simulink model "UserPowerTrain"  (R2025a)
settings: Solver=ode1  StartTime=0.0  StopTime=inf  FixedStep=0.001  RelTol=1e-3  EnableMultiTasking=on
undefined symbols (not defined in the file): DiscIntNeverNeededParam
libraries: CarMaker4SL x7
(part 2 of 3)

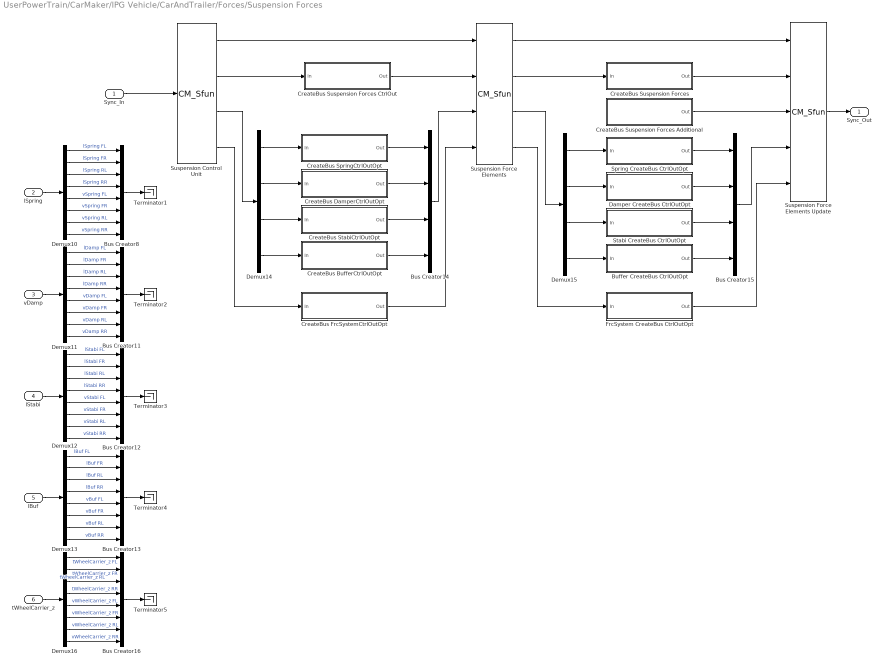
== system UserPowerTrain/CarMaker/IPG Vehicle/CarAndTrailer/Forces/Suspension Forces ==
  Sync_In : Inport
  lSpring : Inport  Port=2
  vDamp : Inport  Port=3
  lStabi : Inport  Port=4
  lBuf : Inport  Port=5
  tWheelCarrier_z : Inport  Port=6
  Buffer CreateBus CtrlOutOpt : Subsystem
  Bus Creator{8,11..13,16} (5 alike) : BusCreator  Inputs=8
  Bus Creator14 : BusCreator  Inputs=4
  Bus Creator15 : BusCreator  Inputs=4
  CreateBus BufferCtrlOutOpt : Subsystem
  CreateBus DamperCtrlOutOpt : Subsystem
  CreateBus FrcSystemCtrlOutOpt : Subsystem
  CreateBus SpringCtrlOutOpt : Subsystem
  CreateBus StabiCtrlOutOpt : Subsystem
  CreateBus Suspension Forces : Subsystem
  CreateBus Suspension Forces Additional : Subsystem
  CreateBus Suspension Forces CtrlOut : Subsystem
  Damper CreateBus CtrlOutOpt : Subsystem
  Demux{10..13,16} (5 alike) : Demux  Outputs=8
      settings: DisplayOption=none
  Demux14 : Demux
      settings: DisplayOption=none
  Demux15 : Demux
      settings: DisplayOption=none
  FrcSystem CreateBus CtrlOutOpt : Subsystem
  Spring CreateBus CtrlOutOpt : Subsystem
  Stabi CreateBus CtrlOutOpt : Subsystem
  Suspension Control Unit : S-Function  FunctionName=CM_Sfun  Parameters='ForcesSuspControl'  SFunctionDeploymentMode=off  EnableBusSupport=off
  Suspension Force Elements : S-Function  FunctionName=CM_Sfun  Parameters='ForcesSusp'  SFunctionDeploymentMode=off  EnableBusSupport=off
  Suspension Force Elements Update : S-Function  FunctionName=CM_Sfun  Parameters='ForcesSuspUpd'  SFunctionDeploymentMode=off  EnableBusSupport=off
  Terminator{1..5} (5 alike) : Terminator
  Sync_Out : Outport  VectorParamsAs1DForOutWhenUnconnected=off
  wires:
  Sync_In/1 -> Suspension Control Unit/1
  Suspension Control Unit/1 -> Suspension Force Elements/1
  Suspension Force Elements/1 -> Suspension Force Elements Update/1
  Suspension Force Elements Update/1 -> Sync_Out/1
  Demux13/4 -> Bus Creator13/4  "lBuf RR"
  Demux11/2 -> Bus Creator11/2  "lDamp FR"
  Demux13/8 -> Bus Creator13/8  "vBuf RR"
  Demux10/3 -> Bus Creator8/3  "lSpring RL"
  Demux10/1 -> Bus Creator8/1  "lSpring FL"
  vDamp/1 -> Demux11/1
  Demux13/2 -> Bus Creator13/2  "lBuf FR"
  Demux10/5 -> Bus Creator8/5  "vSpring FL"
  Bus Creator12/1 -> Terminator3/1
  Demux12/7 -> Bus Creator12/7  "vStabi RL"
  Demux10/4 -> Bus Creator8/4  "lSpring RR"
  Demux12/2 -> Bus Creator12/2  "lStabi FR"
  Demux11/5 -> Bus Creator11/5  "vDamp FL"
  Demux10/8 -> Bus Creator8/8  "vSpring RR"
  Demux12/1 -> Bus Creator12/1  "lStabi FL"
  Demux12/3 -> Bus Creator12/3  "lStabi RL"
  Demux11/6 -> Bus Creator11/6  "vDamp FR"
  lSpring/1 -> Demux10/1
  lBuf/1 -> Demux13/1
  Demux12/4 -> Bus Creator12/4  "lStabi RR"
  Bus Creator13/1 -> Terminator4/1
  Demux13/7 -> Bus Creator13/7  "vBuf RL"
  Demux12/8 -> Bus Creator12/8  "vStabi RR"
  Demux10/7 -> Bus Creator8/7  "vSpring RL"
  Demux11/8 -> Bus Creator11/8  "vDamp RR"
  Demux12/6 -> Bus Creator12/6  "vStabi FR"
  Demux11/1 -> Bus Creator11/1  "lDamp FL"
  Demux11/7 -> Bus Creator11/7  "vDamp RL"
  lStabi/1 -> Demux12/1
  Demux12/5 -> Bus Creator12/5  "vStabi FL"
  Bus Creator8/1 -> Terminator1/1
  Bus Creator11/1 -> Terminator2/1
  Demux13/1 -> Bus Creator13/1  "lBuf FL"
  Demux13/6 -> Bus Creator13/6  "vBuf FR"
  Demux11/4 -> Bus Creator11/4  "lDamp RR"
  Demux13/5 -> Bus Creator13/5  "vBuf FL"
  Demux10/6 -> Bus Creator8/6  "vSpring FR"
  Demux11/3 -> Bus Creator11/3  "lDamp RL"
  Demux10/2 -> Bus Creator8/2  "lSpring FR"
  Demux13/3 -> Bus Creator13/3  "lBuf RL"
  Suspension Force Elements/4 -> FrcSystem CreateBus CtrlOutOpt/1(In)
  FrcSystem CreateBus CtrlOutOpt/1(Out) -> Suspension Force Elements Update/5
  CreateBus SpringCtrlOutOpt/1(Out) -> Bus Creator14/1
  Demux14/1 -> CreateBus SpringCtrlOutOpt/1(In)
  Demux14/2 -> CreateBus DamperCtrlOutOpt/1(In)
  CreateBus DamperCtrlOutOpt/1(Out) -> Bus Creator14/2
  Demux14/3 -> CreateBus StabiCtrlOutOpt/1(In)
  CreateBus StabiCtrlOutOpt/1(Out) -> Bus Creator14/3
  CreateBus BufferCtrlOutOpt/1(Out) -> Bus Creator14/4
  Demux14/4 -> CreateBus BufferCtrlOutOpt/1(In)
  Demux15/4 -> Buffer CreateBus CtrlOutOpt/1(In)
  Buffer CreateBus CtrlOutOpt/1(Out) -> Bus Creator15/4
  Demux15/3 -> Stabi CreateBus CtrlOutOpt/1(In)
  Stabi CreateBus CtrlOutOpt/1(Out) -> Bus Creator15/3
  Demux15/2 -> Damper CreateBus CtrlOutOpt/1(In)
  Damper CreateBus CtrlOutOpt/1(Out) -> Bus Creator15/2
  Demux15/1 -> Spring CreateBus CtrlOutOpt/1(In)
  Spring CreateBus CtrlOutOpt/1(Out) -> Bus Creator15/1
  Suspension Force Elements/3 -> Demux15/1
  Bus Creator15/1 -> Suspension Force Elements Update/4
  Demux16/1 -> Bus Creator16/1  "tWheelCarrier_z FL"
  Demux16/6 -> Bus Creator16/6  "vWheelCarrier_z FR"
  Bus Creator16/1 -> Terminator5/1
  Demux16/2 -> Bus Creator16/2  "tWheelCarrier_z FR"
  Demux16/4 -> Bus Creator16/4  "tWheelCarrier_z RR"
  Demux16/8 -> Bus Creator16/8  "vWheelCarrier_z RR"
  Demux16/7 -> Bus Creator16/7  "vWheelCarrier_z RL"
  Demux16/3 -> Bus Creator16/3  "tWheelCarrier_z RL"
  Demux16/5 -> Bus Creator16/5  "vWheelCarrier_z FL"
  tWheelCarrier_z/1 -> Demux16/1
  CreateBus Suspension Forces Additional/1(Out) -> Suspension Force Elements Update/3
  Suspension Force Elements/2 -> CreateBus Suspension Forces/1(In)
  CreateBus Suspension Forces/1(Out) -> Suspension Force Elements Update/2
  Suspension Control Unit/2 -> CreateBus Suspension Forces CtrlOut/1(In)
  Suspension Control Unit/3 -> Demux14/1
  Suspension Control Unit/4 -> CreateBus FrcSystemCtrlOutOpt/1(In)
  CreateBus FrcSystemCtrlOutOpt/1(Out) -> Suspension Force Elements/4
  Bus Creator14/1 -> Suspension Force Elements/3
  CreateBus Suspension Forces CtrlOut/1(Out) -> Suspension Force Elements/2

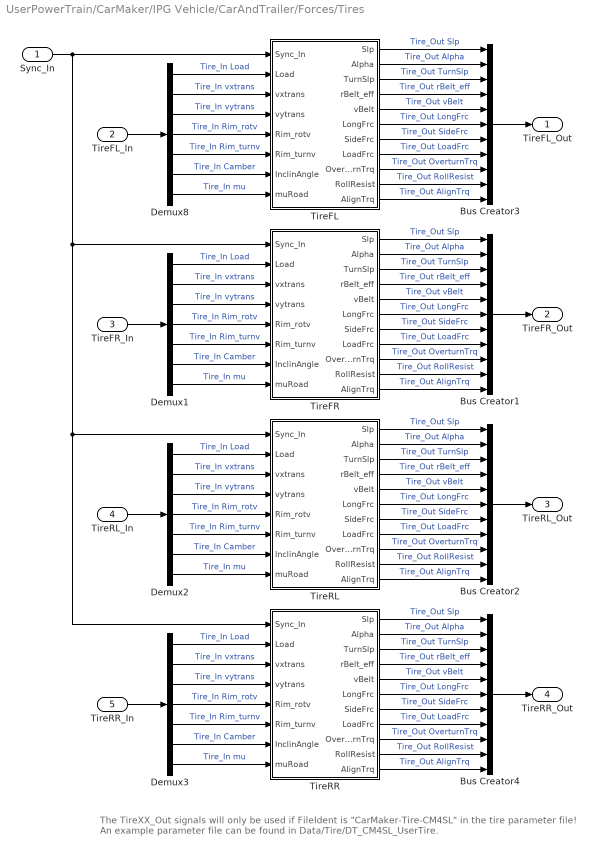
== system UserPowerTrain/CarMaker/IPG Vehicle/CarAndTrailer/Forces/Tires ==
  note: The TireXX_Out signals will only be used if FileIdent is "CarMaker-Tire-CM4SL" in the tire parameter file!
      | An example parameter file can be found in Data/Tire/DT_CM4SL_UserTire.
  Sync_In : Inport
  TireFL_In : Inport  Port=2
  TireFR_In : Inport  Port=3
  TireRL_In : Inport  Port=4
  TireRR_In : Inport  Port=5
  Bus Creator{1..4} (4 alike) : BusCreator  Inputs=11
  Demux{1..3,8} (4 alike) : Demux  Outputs=7
      settings: DisplayOption=none
  TireFL : Subsystem
  TireFR : Subsystem
  TireRL : Subsystem
  TireRR : Subsystem
  TireFL_Out : Outport  VectorParamsAs1DForOutWhenUnconnected=off
  TireFR_Out : Outport  Port=2  VectorParamsAs1DForOutWhenUnconnected=off
  TireRL_Out : Outport  Port=3  VectorParamsAs1DForOutWhenUnconnected=off
  TireRR_Out : Outport  Port=4  VectorParamsAs1DForOutWhenUnconnected=off
  wires:
  Sync_In/1 -> TireRR/1(Sync_In), TireRL/1(Sync_In), TireFR/1(Sync_In), TireFL/1(Sync_In)
  Bus Creator4/1 -> TireRR_Out/1
  Bus Creator2/1 -> TireRL_Out/1
  Bus Creator1/1 -> TireFR_Out/1
  Demux3/5 -> TireRR/6(Rim_turnv)  "Tire_In Rim_turnv"
  Demux3/4 -> TireRR/5(Rim_rotv)  "Tire_In Rim_rotv"
  Demux3/1 -> TireRR/2(Load)  "Tire_In Load"
  Demux3/7 -> TireRR/8(muRoad)  "Tire_In mu"
  Demux3/6 -> TireRR/7(InclinAngle)  "Tire_In Camber"
  Demux3/2 -> TireRR/3(vxtrans)  "Tire_In vxtrans"
  Demux3/3 -> TireRR/4(vytrans)  "Tire_In vytrans"
  TireRR/11(AlignTrq) -> Bus Creator4/11  "Tire_Out AlignTrq"
  TireRR/10(RollResist) -> Bus Creator4/10  "Tire_Out RollResist"
  TireRR/9(OverturnTrq) -> Bus Creator4/9  "Tire_Out OverturnTrq"
  TireRR/8(LoadFrc) -> Bus Creator4/8  "Tire_Out LoadFrc"
  TireRR/7(SideFrc) -> Bus Creator4/7  "Tire_Out SideFrc"
  TireRR/6(LongFrc) -> Bus Creator4/6  "Tire_Out LongFrc"
  TireRR/5(vBelt) -> Bus Creator4/5  "Tire_Out vBelt"
  TireRR/4(rBelt_eff) -> Bus Creator4/4  "Tire_Out rBelt_eff"
  TireRR/3(TurnSlp) -> Bus Creator4/3  "Tire_Out TurnSlp"
  TireRR/1(Slp) -> Bus Creator4/1  "Tire_Out Slp"
  TireRR/2(Alpha) -> Bus Creator4/2  "Tire_Out Alpha"
  Demux2/5 -> TireRL/6(Rim_turnv)  "Tire_In Rim_turnv"
  Demux2/4 -> TireRL/5(Rim_rotv)  "Tire_In Rim_rotv"
  Demux2/1 -> TireRL/2(Load)  "Tire_In Load"
  Demux2/7 -> TireRL/8(muRoad)  "Tire_In mu"
  Demux2/6 -> TireRL/7(InclinAngle)  "Tire_In Camber"
  Demux2/2 -> TireRL/3(vxtrans)  "Tire_In vxtrans"
  Demux2/3 -> TireRL/4(vytrans)  "Tire_In vytrans"
  TireRL/11(AlignTrq) -> Bus Creator2/11  "Tire_Out AlignTrq"
  TireRL/10(RollResist) -> Bus Creator2/10  "Tire_Out RollResist"
  TireRL/9(OverturnTrq) -> Bus Creator2/9  "Tire_Out OverturnTrq"
  TireRL/8(LoadFrc) -> Bus Creator2/8  "Tire_Out LoadFrc"
  TireRL/7(SideFrc) -> Bus Creator2/7  "Tire_Out SideFrc"
  TireRL/6(LongFrc) -> Bus Creator2/6  "Tire_Out LongFrc"
  TireRL/5(vBelt) -> Bus Creator2/5  "Tire_Out vBelt"
  TireRL/4(rBelt_eff) -> Bus Creator2/4  "Tire_Out rBelt_eff"
  TireRL/3(TurnSlp) -> Bus Creator2/3  "Tire_Out TurnSlp"
  TireRL/1(Slp) -> Bus Creator2/1  "Tire_Out Slp"
  TireRL/2(Alpha) -> Bus Creator2/2  "Tire_Out Alpha"
  Demux1/5 -> TireFR/6(Rim_turnv)  "Tire_In Rim_turnv"
  Demux1/4 -> TireFR/5(Rim_rotv)  "Tire_In Rim_rotv"
  Demux1/1 -> TireFR/2(Load)  "Tire_In Load"
  Demux1/7 -> TireFR/8(muRoad)  "Tire_In mu"
  Demux1/6 -> TireFR/7(InclinAngle)  "Tire_In Camber"
  Demux1/2 -> TireFR/3(vxtrans)  "Tire_In vxtrans"
  Demux1/3 -> TireFR/4(vytrans)  "Tire_In vytrans"
  TireFR/11(AlignTrq) -> Bus Creator1/11  "Tire_Out AlignTrq"
  TireFR/10(RollResist) -> Bus Creator1/10  "Tire_Out RollResist"
  TireFR/9(OverturnTrq) -> Bus Creator1/9  "Tire_Out OverturnTrq"
  TireFR/8(LoadFrc) -> Bus Creator1/8  "Tire_Out LoadFrc"
  TireFR/7(SideFrc) -> Bus Creator1/7  "Tire_Out SideFrc"
  TireFR/6(LongFrc) -> Bus Creator1/6  "Tire_Out LongFrc"
  TireFR/5(vBelt) -> Bus Creator1/5  "Tire_Out vBelt"
  TireFR/4(rBelt_eff) -> Bus Creator1/4  "Tire_Out rBelt_eff"
  TireFR/3(TurnSlp) -> Bus Creator1/3  "Tire_Out TurnSlp"
  TireFR/1(Slp) -> Bus Creator1/1  "Tire_Out Slp"
  TireFR/2(Alpha) -> Bus Creator1/2  "Tire_Out Alpha"
  Demux8/5 -> TireFL/6(Rim_turnv)  "Tire_In Rim_turnv"
  Demux8/4 -> TireFL/5(Rim_rotv)  "Tire_In Rim_rotv"
  TireFL_In/1 -> Demux8/1
  Demux8/1 -> TireFL/2(Load)  "Tire_In Load"
  Demux8/7 -> TireFL/8(muRoad)  "Tire_In mu"
  Demux8/6 -> TireFL/7(InclinAngle)  "Tire_In Camber"
  Demux8/2 -> TireFL/3(vxtrans)  "Tire_In vxtrans"
  Demux8/3 -> TireFL/4(vytrans)  "Tire_In vytrans"
  TireFL/11(AlignTrq) -> Bus Creator3/11  "Tire_Out AlignTrq"
  TireFL/10(RollResist) -> Bus Creator3/10  "Tire_Out RollResist"
  TireFL/9(OverturnTrq) -> Bus Creator3/9  "Tire_Out OverturnTrq"
  TireFL/8(LoadFrc) -> Bus Creator3/8  "Tire_Out LoadFrc"
  TireFL/7(SideFrc) -> Bus Creator3/7  "Tire_Out SideFrc"
  TireFL/6(LongFrc) -> Bus Creator3/6  "Tire_Out LongFrc"
  TireFL/5(vBelt) -> Bus Creator3/5  "Tire_Out vBelt"
  TireFL/4(rBelt_eff) -> Bus Creator3/4  "Tire_Out rBelt_eff"
  TireFL/3(TurnSlp) -> Bus Creator3/3  "Tire_Out TurnSlp"
  TireFL/1(Slp) -> Bus Creator3/1  "Tire_Out Slp"
  TireFL/2(Alpha) -> Bus Creator3/2  "Tire_Out Alpha"
  Bus Creator3/1 -> TireFL_Out/1
  TireFR_In/1 -> Demux1/1
  TireRL_In/1 -> Demux2/1
  TireRR_In/1 -> Demux3/1

== system UserPowerTrain/CarMaker/IPG Vehicle/CarAndTrailer/Forces/Vehicle Forces ==
  Sync_In : Inport
  Bus Creator1 : BusCreator  Inputs=12
  Bus Creator8 : BusCreator  Inputs=16
  BusCreator1 : BusCreator  Inputs=4
  BusCreator2 : BusCreator  Inputs=9
  Demux : Demux  Outputs=16
      settings: DisplayOption=none
  Demux1 : Demux  Outputs=12
      settings: DisplayOption=none
  Demux2 : Demux  Outputs=13
      settings: DisplayOption=none
  Forces : S-Function  FunctionName=CM_Sfun  Parameters='Forces'  SFunctionDeploymentMode=off  EnableBusSupport=off
  Terminator : Terminator
  Sync_Out : Outport  VectorParamsAs1DForOutWhenUnconnected=off
  Car.Virtual : Outport  Port=2  VectorParamsAs1DForOutWhenUnconnected=off
  Car.Aero : Outport  Port=3  VectorParamsAs1DForOutWhenUnconnected=off
  Car.Load : Outport  Port=4  VectorParamsAs1DForOutWhenUnconnected=off
  wires:
  BusCreator1/1 -> Terminator/1  "Aero IF (in)"
  Demux2/13 -> BusCreator2/9  "car Aero Trq_1 z"
  Demux2/12 -> BusCreator2/8  "car Aero Trq_1 y"
  Demux2/11 -> BusCreator2/7  "car Aero Trq_1 x"
  Demux2/10 -> BusCreator2/6  "car Aero Frc_1 z"
  Demux2/9 -> BusCreator2/5  "car Aero Frc_1 y"
  Demux2/8 -> BusCreator2/4  "car Aero Frc_1 x"
  Demux2/7 -> BusCreator2/3  "car Aero PoA_1 z"
  Demux2/6 -> BusCreator2/2  "car Aero PoA_1 y"
  Demux2/5 -> BusCreator2/1  "car Aero PoA_1 x"
  Demux2/4 -> BusCreator1/4  "car Aero tau_1"
  Demux2/3 -> BusCreator1/3  "car Aero ApproachVel_1 z"
  Demux2/2 -> BusCreator1/2  "car Aero ApproachVel_1 y"
  Demux2/1 -> BusCreator1/1  "car Aero ApproachVel_1 x"
  Demux/16 -> Bus Creator8/16  "Car Load_3 tz"
  Demux/15 -> Bus Creator8/15  "Car Load_3 ty"
  Demux/14 -> Bus Creator8/14  "Car Load_3 tx"
  Demux/13 -> Bus Creator8/13  "Car Load_3 mass"
  Demux1/12 -> Bus Creator1/12  "Car Virtual Trq_0 z"
  Demux1/11 -> Bus Creator1/11  "Car Virtual Trq_0 y"
  Demux1/10 -> Bus Creator1/10  "Car Virtual Trq_0 x"
  Demux1/9 -> Bus Creator1/9  "Car Virtual Trq_1 z"
  Demux1/8 -> Bus Creator1/8  "Car Virtual Trq_1 y"
  Demux1/7 -> Bus Creator1/7  "Car Virtual Trq_1 x"
  Demux1/6 -> Bus Creator1/6  "Car Virtual Frc_0 z"
  Demux1/5 -> Bus Creator1/5  "Car Virtual Frc_0 y"
  Demux1/4 -> Bus Creator1/4  "Car Virtual Frc_0 x"
  Sync_In/1 -> Forces/1
  Forces/1 -> Sync_Out/1
  BusCreator2/1 -> Car.Aero/1
  Demux1/1 -> Bus Creator1/1  "Car Virtual Frc_1 x"
  Demux1/2 -> Bus Creator1/2  "Car Virtual Frc_1 y"
  Demux1/3 -> Bus Creator1/3  "Car Virtual Frc_1 z"
  Forces/3 -> Demux2/1
  Forces/2 -> Demux1/1
  Bus Creator1/1 -> Car.Virtual/1
  Bus Creator8/1 -> Car.Load/1
  Demux/1 -> Bus Creator8/1  "Car Load_0 mass"
  Demux/2 -> Bus Creator8/2  "Car Load_0 tx"
  Demux/3 -> Bus Creator8/3  "Car Load_0 ty"
  Demux/4 -> Bus Creator8/4  "Car Load_0 tz"
  Demux/5 -> Bus Creator8/5  "Car Load_1 mass"
  Demux/6 -> Bus Creator8/6  "Car Load_1 tx"
  Demux/7 -> Bus Creator8/7  "Car Load_1 ty"
  Demux/8 -> Bus Creator8/8  "Car Load_1 tz"
  Demux/9 -> Bus Creator8/9  "Car Load_2 mass"
  Demux/10 -> Bus Creator8/10  "Car Load_2 tx"
  Demux/11 -> Bus Creator8/11  "Car Load_2 ty"
  Demux/12 -> Bus Creator8/12  "Car Load_2 tz"
  Forces/4 -> Demux/1

== system UserPowerTrain/CarMaker/IPG Vehicle/CarAndTrailer/Trailer/CreateBus Car.Hitch.FrcTrq ==
  In1 : Inport
  Bus Creator7 : BusCreator  Inputs=6
  Demux7 : Demux  Outputs=6
      settings: DisplayOption=none
  Out1 : Outport  VectorParamsAs1DForOutWhenUnconnected=off
  wires:
  In1/1 -> Demux7/1
  Bus Creator7/1 -> Out1/1
  Demux7/6 -> Bus Creator7/6  "Car Hitch Trq2Car z"
  Demux7/5 -> Bus Creator7/5  "Car Hitch Trq2Car y"
  Demux7/4 -> Bus Creator7/4  "Car Hitch Trq2Car x"
  Demux7/3 -> Bus Creator7/3  "Car Hitch Frc2Car z"
  Demux7/2 -> Bus Creator7/2  "Car Hitch Frc2Car y"
  Demux7/1 -> Bus Creator7/1  "Car Hitch Frc2Car x"

== system UserPowerTrain/CarMaker/IPG Vehicle/CarAndTrailer/Trailer/CreateBus Vhcl.Motion ==
  In1 : Inport
  BusCreator : BusCreator  Inputs=15
  Demux : Demux  Outputs=15
      settings: DisplayOption=none
  Out1 : Outport  VectorParamsAs1DForOutWhenUnconnected=off
  wires:
  Demux/15 -> BusCreator/15  "Vhcl YawAcc"
  Demux/14 -> BusCreator/14  "Vhcl YawVel"
  Demux/13 -> BusCreator/13  "Vhcl Yaw"
  Demux/12 -> BusCreator/12  "Vhcl PitchAcc"
  Demux/11 -> BusCreator/11  "Vhcl PitchVel"
  Demux/10 -> BusCreator/10  "Vhcl Pitch"
  Demux/9 -> BusCreator/9  "Vhcl RollAcc"
  Demux/8 -> BusCreator/8  "Vhcl RollVel"
  Demux/7 -> BusCreator/7  "Vhcl Roll"
  Demux/6 -> BusCreator/6  "Vhcl Hitch_Pos z"
  Demux/5 -> BusCreator/5  "Vhcl Hitch_Pos y"
  Demux/4 -> BusCreator/4  "Vhcl Hitch_Pos x"
  Demux/3 -> BusCreator/3  "Vhcl sRoad"
  Demux/2 -> BusCreator/2  "Vhcl Distance"
  Demux/1 -> BusCreator/1  "Vhcl v"
  In1/1 -> Demux/1
  BusCreator/1 -> Out1/1

== system UserPowerTrain/CarMaker/IPG Vehicle/CarAndTrailer/Trailer/CreateBus Vhcl.PoI ==
  In1 : Inport
  Bus Creator3 : BusCreator  Inputs=18
  Demux3 : Demux  Outputs=18
      settings: DisplayOption=none
  Out1 : Outport  VectorParamsAs1DForOutWhenUnconnected=off
  wires:
  Demux3/18 -> Bus Creator3/18  "Vhcl PoI_GCS Elev"
  Demux3/17 -> Bus Creator3/17  "Vhcl PoI_GCS Lat"
  Demux3/16 -> Bus Creator3/16  "Vhcl PoI_GCS Long"
  Demux3/15 -> Bus Creator3/15  "Vhcl PoI_Acc_1 z"
  Demux3/14 -> Bus Creator3/14  "Vhcl PoI_Acc_1 y"
  Demux3/13 -> Bus Creator3/13  "Vhcl PoI_Acc_1 x"
  Demux3/12 -> Bus Creator3/12  "Vhcl PoI_Vel_1 z"
  Demux3/11 -> Bus Creator3/11  "Vhcl PoI_Vel_1 y"
  Demux3/10 -> Bus Creator3/10  "Vhcl PoI_Vel_1 x"
  Demux3/9 -> Bus Creator3/9  "Vhcl PoI_Acc z"
  Demux3/8 -> Bus Creator3/8  "Vhcl PoI_Acc y"
  Demux3/7 -> Bus Creator3/7  "Vhcl PoI_Acc x"
  Demux3/6 -> Bus Creator3/6  "Vhcl PoI_Vel z"
  Demux3/5 -> Bus Creator3/5  "Vhcl PoI_Vel y"
  Demux3/4 -> Bus Creator3/4  "Vhcl PoI_Vel x"
  Demux3/3 -> Bus Creator3/3  "Vhcl PoI_Pos z"
  Demux3/2 -> Bus Creator3/2  "Vhcl PoI_Pos y"
  In1/1 -> Demux3/1
  Bus Creator3/1 -> Out1/1
  Demux3/1 -> Bus Creator3/1  "Vhcl PoI_Pos x"

== system UserPowerTrain/CarMaker/IPG Vehicle/CarAndTrailer/Trailer/CreateBus Vhcl.Steering ==
  In1 : Inport
  Bus Creator3 : BusCreator  Inputs=4
  Demux : Demux
      settings: DisplayOption=none
  Out1 : Outport  VectorParamsAs1DForOutWhenUnconnected=off
  wires:
  Bus Creator3/1 -> Out1/1
  Demux/1 -> Bus Creator3/1  "Vhcl Steering Ang"
  Demux/3 -> Bus Creator3/3  "Vhcl Steering AngAcc"
  Demux/2 -> Bus Creator3/2  "Vhcl Steering AngVel"
  Demux/4 -> Bus Creator3/4  "Vhcl Steering Trq"
  In1/1 -> Demux/1

== system UserPowerTrain/CarMaker/IPG Vehicle/CarAndTrailer/Trailer/CreateBus Vhcl.Wheel.FL ==
  In1 : Inport
  Bus Creator3 : BusCreator  Inputs=14
  Demux3 : Demux  Outputs=14
      settings: DisplayOption=none
  Out1 : Outport  VectorParamsAs1DForOutWhenUnconnected=off
  wires:
  Demux3/14 -> Bus Creator3/14  "Vhcl Wheel FL Trq_WhlBearing"
  Demux3/13 -> Bus Creator3/13  "Vhcl Wheel FL Trq_T2W"
  Demux3/12 -> Bus Creator3/12  "Vhcl Wheel FL SideSlip"
  Demux3/11 -> Bus Creator3/11  "Vhcl Wheel FL LongSlip"
  Demux3/10 -> Bus Creator3/10  "Vhcl Wheel FL vBelt"
  Demux3/9 -> Bus Creator3/9  "Vhcl Wheel FL Fz"
  Demux3/8 -> Bus Creator3/8  "Vhcl Wheel FL Fy"
  Demux3/7 -> Bus Creator3/7  "Vhcl Wheel FL Fx"
  Demux3/6 -> Bus Creator3/6  "Vhcl Wheel FL r_zxy z"
  Demux3/5 -> Bus Creator3/5  "Vhcl Wheel FL r_zxy y"
  Demux3/4 -> Bus Creator3/4  "Vhcl Wheel FL r_zxy x"
  Demux3/3 -> Bus Creator3/3  "Vhcl Wheel FL t z"
  Demux3/2 -> Bus Creator3/2  "Vhcl Wheel FL t y"
  In1/1 -> Demux3/1
  Bus Creator3/1 -> Out1/1
  Demux3/1 -> Bus Creator3/1  "Vhcl Wheel FL t x"

== system UserPowerTrain/CarMaker/IPG Vehicle/CarAndTrailer/Trailer/CreateBus Vhcl.Wheel.FR ==
  In1 : Inport
  Bus Creator3 : BusCreator  Inputs=14
  Demux3 : Demux  Outputs=14
      settings: DisplayOption=none
  Out1 : Outport  VectorParamsAs1DForOutWhenUnconnected=off
  wires:
  Demux3/14 -> Bus Creator3/14  "Vhcl Wheel FR Trq_WhlBearing"
  Demux3/13 -> Bus Creator3/13  "Vhcl Wheel FR Trq_T2W"
  Demux3/12 -> Bus Creator3/12  "Vhcl Wheel FR SideSlip"
  Demux3/11 -> Bus Creator3/11  "Vhcl Wheel FR LongSlip"
  Demux3/10 -> Bus Creator3/10  "Vhcl Wheel FR vBelt"
  Demux3/9 -> Bus Creator3/9  "Vhcl Wheel FR Fz"
  Demux3/8 -> Bus Creator3/8  "Vhcl Wheel FR Fy"
  Demux3/7 -> Bus Creator3/7  "Vhcl Wheel FR Fx"
  Demux3/6 -> Bus Creator3/6  "Vhcl Wheel FR r_zxy z"
  Demux3/5 -> Bus Creator3/5  "Vhcl Wheel FR r_zxy y"
  Demux3/4 -> Bus Creator3/4  "Vhcl Wheel FR r_zxy x"
  Demux3/3 -> Bus Creator3/3  "Vhcl Wheel FR t z"
  Demux3/2 -> Bus Creator3/2  "Vhcl Wheel FR t y"
  In1/1 -> Demux3/1
  Bus Creator3/1 -> Out1/1
  Demux3/1 -> Bus Creator3/1  "Vhcl Wheel FR t x"

== system UserPowerTrain/CarMaker/IPG Vehicle/CarAndTrailer/Trailer/CreateBus Vhcl.Wheel.RL ==
  In1 : Inport
  Bus Creator3 : BusCreator  Inputs=14
  Demux3 : Demux  Outputs=14
      settings: DisplayOption=none
  Out1 : Outport  VectorParamsAs1DForOutWhenUnconnected=off
  wires:
  Demux3/14 -> Bus Creator3/14  "Vhcl Wheel RL Trq_WhlBearing"
  Demux3/13 -> Bus Creator3/13  "Vhcl Wheel RL Trq_T2W"
  Demux3/12 -> Bus Creator3/12  "Vhcl Wheel RL SideSlip"
  Demux3/11 -> Bus Creator3/11  "Vhcl Wheel RL LongSlip"
  Demux3/10 -> Bus Creator3/10  "Vhcl Wheel RL vBelt"
  Demux3/9 -> Bus Creator3/9  "Vhcl Wheel RL Fz"
  Demux3/8 -> Bus Creator3/8  "Vhcl Wheel RL Fy"
  Demux3/7 -> Bus Creator3/7  "Vhcl Wheel RL Fx"
  Demux3/6 -> Bus Creator3/6  "Vhcl Wheel RL r_zxy z"
  Demux3/5 -> Bus Creator3/5  "Vhcl Wheel RL r_zxy y"
  Demux3/4 -> Bus Creator3/4  "Vhcl Wheel RL r_zxy x"
  Demux3/3 -> Bus Creator3/3  "Vhcl Wheel RL t z"
  Demux3/2 -> Bus Creator3/2  "Vhcl Wheel RL t y"
  In1/1 -> Demux3/1
  Bus Creator3/1 -> Out1/1
  Demux3/1 -> Bus Creator3/1  "Vhcl Wheel RL t x"

== system UserPowerTrain/CarMaker/IPG Vehicle/CarAndTrailer/Trailer/CreateBus Vhcl.Wheel.RR ==
  In1 : Inport
  Bus Creator3 : BusCreator  Inputs=14
  Demux3 : Demux  Outputs=14
      settings: DisplayOption=none
  Out1 : Outport  VectorParamsAs1DForOutWhenUnconnected=off
  wires:
  Demux3/14 -> Bus Creator3/14  "Vhcl Wheel RR Trq_WhlBearing"
  Demux3/13 -> Bus Creator3/13  "Vhcl Wheel RR Trq_T2W"
  Demux3/12 -> Bus Creator3/12  "Vhcl Wheel RR SideSlip"
  Demux3/11 -> Bus Creator3/11  "Vhcl Wheel RR LongSlip"
  Demux3/10 -> Bus Creator3/10  "Vhcl Wheel RR vBelt"
  Demux3/9 -> Bus Creator3/9  "Vhcl Wheel RR Fz"
  Demux3/8 -> Bus Creator3/8  "Vhcl Wheel RR Fy"
  Demux3/7 -> Bus Creator3/7  "Vhcl Wheel RR Fx"
  Demux3/6 -> Bus Creator3/6  "Vhcl Wheel RR r_zxy z"
  Demux3/5 -> Bus Creator3/5  "Vhcl Wheel RR r_zxy y"
  Demux3/4 -> Bus Creator3/4  "Vhcl Wheel RR r_zxy x"
  Demux3/3 -> Bus Creator3/3  "Vhcl Wheel RR t z"
  Demux3/2 -> Bus Creator3/2  "Vhcl Wheel RR t y"
  In1/1 -> Demux3/1
  Bus Creator3/1 -> Out1/1
  Demux3/1 -> Bus Creator3/1  "Vhcl Wheel RR t x"

== system UserPowerTrain/CarMaker/IPG Vehicle/PowerTrain/User RearDriven PowerTrain/Diff Trq ==
  In1 : Inport
  Gain10 : Gain  Gain=0.5
  Product : Product  RndMeth=Zero
  Read CM Parameter : CarMaker4SL/Read CM Parameter  xfile_type=Vehicle  xfile_instance_vehicle=-  xfile_instance_trailer=1  xfile_instance_general=-  xfile_kind_vehicle=Vehicle  xfile_kind_trailer=Trailer  xfile_kind_general=SimParameters  xfile=Vehicle  xkey=PowerTrain.DL.iDiff  xnout=1  xdefaults=[]  xmuxed=on  xstime=Continuous
      settings: SourceProductName=CarMaker4SL
  Out1 : Outport  VectorParamsAs1DForOutWhenUnconnected=off
  wires:
  Gain10/1 -> Out1/1
  Read CM Parameter/1 -> Product/1
  In1/1 -> Product/2
  Product/1 -> Gain10/1  "DiffTrq"

== system UserPowerTrain/CarMaker/IPG Vehicle/PowerTrain/User RearDriven PowerTrain/Diff rotv ==
  In1 : Inport
  In2 : Inport  Port=2
  Gain11 : Gain  Gain=1/2
  Memory : Memory
  Memory1 : Memory
  Product : Product  RndMeth=Zero
  Read CM Parameter : CarMaker4SL/Read CM Parameter  xfile_type=Vehicle  xfile_instance_vehicle=-  xfile_instance_trailer=1  xfile_instance_general=-  xfile_kind_vehicle=Vehicle  xfile_kind_trailer=Trailer  xfile_kind_general=SimParameters  xfile=Vehicle  xkey=PowerTrain.DL.iDiff  xnout=1  xdefaults=[]  xmuxed=on  xstime=Continuous
      settings: SourceProductName=CarMaker4SL
  Sum2 : Sum  Inputs=|++
  Out1 : Outport  VectorParamsAs1DForOutWhenUnconnected=off
  wires:
  Gain11/1 -> Product/2
  In2/1 -> Memory1/1
  Sum2/1 -> Gain11/1
  Memory1/1 -> Sum2/2
  Memory/1 -> Sum2/1
  Read CM Parameter/1 -> Product/1
  In1/1 -> Memory/1
  Product/1 -> Out1/1  "DiffTrq"

== system UserPowerTrain/CarMaker/IPG Vehicle/PowerTrain/User RearDriven PowerTrain/Engine Trq ==
  Engine rotv : Inport
  Gas : Inport  Port=2
  Lookup Table : Lookup  InputValues=[0 1000 2000 5000 7000]  Table=[0 140 180 200 0]  SaturateOnIntegerOverflow=off
  Product : Product  RndMeth=Zero
  Engine Trq : Outport  VectorParamsAs1DForOutWhenUnconnected=off
  wires:
  Engine rotv/1 -> Lookup Table/1
  Product/1 -> Engine Trq/1
  Gas/1 -> Product/2
  Lookup Table/1 -> Product/1

== system UserPowerTrain/CarMaker/IPG Vehicle/PowerTrain/User RearDriven PowerTrain/GB Trq ==
  In1 : Inport
  In2 : Inport  Port=2
  Product : Product  RndMeth=Zero
  Out1 : Outport  VectorParamsAs1DForOutWhenUnconnected=off
  wires:
  In2/1 -> Product/2
  In1/1 -> Product/1
  Product/1 -> Out1/1  "GearBox Trq"

== system UserPowerTrain/CarMaker/IPG Vehicle/PowerTrain/User RearDriven PowerTrain/GB rotv ==
  In1 : Inport
  In2 : Inport  Port=2
  Product : Product  RndMeth=Zero
  Out1 : Outport  VectorParamsAs1DForOutWhenUnconnected=off
  wires:
  In2/1 -> Product/2
  In1/1 -> Product/1
  Product/1 -> Out1/1

== system UserPowerTrain/CarMaker/IPG Vehicle/PowerTrain/User RearDriven PowerTrain/GearRatio ==
  In2 : Inport
  Product2 : Product  RndMeth=Zero
  Read CM Parameter2 : CarMaker4SL/Read CM Parameter  xfile_type=Vehicle  xfile_instance_vehicle=-  xfile_instance_trailer=1  xfile_instance_general=-  xfile_kind_vehicle=Vehicle  xfile_kind_trailer=Trailer  xfile_kind_general=SimParameters  xfile=Vehicle  xkey=PowerTrain.Gearbox.0.iForwardGears  xnout=5  xdefaults=[]  xmuxed=on  xstime=Continuous
      settings: SourceProductName=CarMaker4SL
  Saturation : Saturate  UpperLimit=5  LowerLimit=1
  Selector : Selector  InputPortWidth=5  IndexOptions=Index vector (port)  Indices=[1 3]  OutputSizes=1
  Sign : Signum
  Out1 : Outport  VectorParamsAs1DForOutWhenUnconnected=off
  wires:
  Sign/1 -> Product2/2
  Product2/1 -> Out1/1
  Selector/1 -> Product2/1
  Saturation/1 -> Selector/2
  In2/1 -> Sign/1, Saturation/1
  Read CM Parameter2/1 -> Selector/1

== system UserPowerTrain/CarMaker/IPG Vehicle/PowerTrain/User RearDriven PowerTrain/WheelInertia ==
  In1 : Inport
  Divide : Product  Inputs=*/
  Read CM Parameter : CarMaker4SL/Read CM Parameter  xfile_type=Vehicle  xfile_instance_vehicle=-  xfile_instance_trailer=1  xfile_instance_general=-  xfile_kind_vehicle=Vehicle  xfile_kind_trailer=Trailer  xfile_kind_general=SimParameters  xfile=Vehicle  xkey=Wheel.fl.I  xnout=3  xdefaults=[]  xmuxed=off  xstime=Continuous
      settings: SourceProductName=CarMaker4SL
  Switch : Switch  Criteria=u2 ~= 0  ZeroCross=off  SaturateOnIntegerOverflow=off  InputSameDT=off
  Terminator : Terminator
  Terminator1 : Terminator
  Zero : Constant
  Out1 : Outport  VectorParamsAs1DForOutWhenUnconnected=off
  wires:
  Read CM Parameter/2 -> Switch/1, Switch/2
  Switch/1 -> Divide/2
  Zero/1 -> Switch/3
  In1/1 -> Divide/1
  Read CM Parameter/3 -> Terminator1/1
  Read CM Parameter/1 -> Terminator/1
  Divide/1 -> Out1/1

== system UserPowerTrain/CarMaker/IPG Vehicle/PowerTrain/User RearDriven PowerTrain/WheelInertia1 ==
  In1 : Inport
  Divide : Product  Inputs=*/
  Read CM Parameter : CarMaker4SL/Read CM Parameter  xfile_type=Vehicle  xfile_instance_vehicle=-  xfile_instance_trailer=1  xfile_instance_general=-  xfile_kind_vehicle=Vehicle  xfile_kind_trailer=Trailer  xfile_kind_general=SimParameters  xfile=Vehicle  xkey=Wheel.fr.I  xnout=3  xdefaults=[]  xmuxed=off  xstime=Continuous
      settings: SourceProductName=CarMaker4SL
  Switch : Switch  Criteria=u2 ~= 0  ZeroCross=off  SaturateOnIntegerOverflow=off  InputSameDT=off
  Terminator : Terminator
  Terminator1 : Terminator
  Zero : Constant
  Out1 : Outport  VectorParamsAs1DForOutWhenUnconnected=off
  wires:
  Divide/1 -> Out1/1
  Read CM Parameter/1 -> Terminator/1
  Read CM Parameter/3 -> Terminator1/1
  In1/1 -> Divide/1
  Read CM Parameter/2 -> Switch/2, Switch/1
  Zero/1 -> Switch/3
  Switch/1 -> Divide/2

== system UserPowerTrain/CarMaker/IPG Vehicle/PowerTrain/User RearDriven PowerTrain/WheelInertia2 ==
  In1 : Inport
  Divide : Product  Inputs=*/
  Read CM Parameter : CarMaker4SL/Read CM Parameter  xfile_type=Vehicle  xfile_instance_vehicle=-  xfile_instance_trailer=1  xfile_instance_general=-  xfile_kind_vehicle=Vehicle  xfile_kind_trailer=Trailer  xfile_kind_general=SimParameters  xfile=Vehicle  xkey=Wheel.rl.I  xnout=3  xdefaults=[]  xmuxed=off  xstime=Continuous
      settings: SourceProductName=CarMaker4SL
  Switch : Switch  Criteria=u2 ~= 0  ZeroCross=off  SaturateOnIntegerOverflow=off  InputSameDT=off
  Terminator : Terminator
  Terminator1 : Terminator
  Zero : Constant
  Out1 : Outport  VectorParamsAs1DForOutWhenUnconnected=off
  wires:
  Switch/1 -> Divide/2
  Zero/1 -> Switch/3
  Read CM Parameter/2 -> Switch/1, Switch/2
  In1/1 -> Divide/1
  Read CM Parameter/3 -> Terminator1/1
  Read CM Parameter/1 -> Terminator/1
  Divide/1 -> Out1/1

== system UserPowerTrain/CarMaker/IPG Vehicle/PowerTrain/User RearDriven PowerTrain/WheelInertia3 ==
  In1 : Inport
  Divide : Product  Inputs=*/
  Read CM Parameter : CarMaker4SL/Read CM Parameter  xfile_type=Vehicle  xfile_instance_vehicle=-  xfile_instance_trailer=1  xfile_instance_general=-  xfile_kind_vehicle=Vehicle  xfile_kind_trailer=Trailer  xfile_kind_general=SimParameters  xfile=Vehicle  xkey=Wheel.rr.I  xnout=3  xdefaults=[]  xmuxed=off  xstime=Continuous
      settings: SourceProductName=CarMaker4SL
  Switch : Switch  Criteria=u2 ~= 0  ZeroCross=off  SaturateOnIntegerOverflow=off  InputSameDT=off
  Terminator : Terminator
  Terminator1 : Terminator
  Zero : Constant
  Out1 : Outport  VectorParamsAs1DForOutWhenUnconnected=off
  wires:
  Divide/1 -> Out1/1
  Read CM Parameter/1 -> Terminator/1
  Read CM Parameter/3 -> Terminator1/1
  In1/1 -> Divide/1
  Read CM Parameter/2 -> Switch/2, Switch/1
  Zero/1 -> Switch/3
  Switch/1 -> Divide/2

== system UserPowerTrain/CarMaker/IPG Vehicle/CarAndTrailer/Forces/Suspension Forces/Buffer CreateBus CtrlOutOpt ==
  note: <Your model here>
  In : Inport
  Bus Creator{,1..3,9} (5 alike) : BusCreator  Inputs=4
  Demux{,2..5} (5 alike) : Demux
  Out : Outport
  wires:
  Bus Creator/1 -> Bus Creator9/1
  Demux/4 -> Demux5/1  "RR"
  Bus Creator2/1 -> Bus Creator9/3
  Demux5/1 -> Bus Creator3/1  "RR CtrlOutOpt0"
  Bus Creator3/1 -> Bus Creator9/4
  Demux2/4 -> Bus Creator/4  "FL CtrlOutOpt3"
  Demux5/3 -> Bus Creator3/3  "RR CtrlOutOpt2"
  Demux4/3 -> Bus Creator2/3  "RL CtrlOutOpt2"
  Bus Creator1/1 -> Bus Creator9/2
  Demux4/2 -> Bus Creator2/2  "RL CtrlOutOpt1"
  Demux2/2 -> Bus Creator/2  "FL CtrlOutOpt1"
  Demux/2 -> Demux3/1  "FR"
  Demux3/4 -> Bus Creator1/4  "FR CtrlOutOpt3"
  Demux3/1 -> Bus Creator1/1  "FR CtrlOutOpt0"
  Demux4/4 -> Bus Creator2/4  "RL CtrlOutOpt3"
  Demux2/3 -> Bus Creator/3  "FL CtrlOutOpt2"
  Demux3/2 -> Bus Creator1/2  "FR CtrlOutOpt1"
  Demux2/1 -> Bus Creator/1  "FL CtrlOutOpt0"
  Demux3/3 -> Bus Creator1/3  "FR CtrlOutOpt2"
  In/1 -> Demux/1
  Demux5/4 -> Bus Creator3/4  "RR CtrlOutOpt3"
  Demux/3 -> Demux4/1  "RL"
  Bus Creator9/1 -> Out/1
  Demux5/2 -> Bus Creator3/2  "RR CtrlOutOpt1"
  Demux4/1 -> Bus Creator2/1  "RL CtrlOutOpt0"
  Demux/1 -> Demux2/1  "FL"

== system UserPowerTrain/CarMaker/IPG Vehicle/CarAndTrailer/Forces/Suspension Forces/CreateBus BufferCtrlOutOpt ==
  note: <Your model here>
  In : Inport
  Bus Creator{,1..3,9} (5 alike) : BusCreator  Inputs=4
  Demux{,2..5} (5 alike) : Demux
  Out : Outport
  wires:
  Bus Creator/1 -> Bus Creator9/1
  Demux/4 -> Demux5/1  "RR"
  Bus Creator2/1 -> Bus Creator9/3
  Demux5/1 -> Bus Creator3/1  "RR CtrlOutOpt0"
  Bus Creator3/1 -> Bus Creator9/4
  Demux2/4 -> Bus Creator/4  "FL CtrlOutOpt3"
  Demux5/3 -> Bus Creator3/3  "RR CtrlOutOpt2"
  Demux4/3 -> Bus Creator2/3  "RL CtrlOutOpt2"
  Bus Creator1/1 -> Bus Creator9/2
  Demux4/2 -> Bus Creator2/2  "RL CtrlOutOpt1"
  Demux2/2 -> Bus Creator/2  "FL CtrlOutOpt1"
  Demux/2 -> Demux3/1  "FR"
  Demux3/4 -> Bus Creator1/4  "FR CtrlOutOpt3"
  Demux3/1 -> Bus Creator1/1  "FR CtrlOutOpt0"
  Demux4/4 -> Bus Creator2/4  "RL CtrlOutOpt3"
  Demux2/3 -> Bus Creator/3  "FL CtrlOutOpt2"
  Demux3/2 -> Bus Creator1/2  "FR CtrlOutOpt1"
  Demux2/1 -> Bus Creator/1  "FL CtrlOutOpt0"
  Demux3/3 -> Bus Creator1/3  "FR CtrlOutOpt2"
  Demux5/4 -> Bus Creator3/4  "RR CtrlOutOpt3"
  Demux/3 -> Demux4/1  "RL"
  Bus Creator9/1 -> Out/1
  Demux5/2 -> Bus Creator3/2  "RR CtrlOutOpt1"
  Demux4/1 -> Bus Creator2/1  "RL CtrlOutOpt0"
  Demux/1 -> Demux2/1  "FL"
  In/1 -> Demux/1

== system UserPowerTrain/CarMaker/IPG Vehicle/CarAndTrailer/Forces/Suspension Forces/CreateBus DamperCtrlOutOpt ==
  note: <Your model here>
  In : Inport
  Bus Creator{,1..3,9} (5 alike) : BusCreator  Inputs=4
  Demux{,2..5} (5 alike) : Demux
  Out : Outport
  wires:
  Bus Creator/1 -> Bus Creator9/1
  Demux/4 -> Demux5/1  "RR"
  Bus Creator2/1 -> Bus Creator9/3
  Demux5/1 -> Bus Creator3/1  "RR CtrlOutOpt0"
  Bus Creator3/1 -> Bus Creator9/4
  Demux2/4 -> Bus Creator/4  "FL CtrlOutOpt3"
  Demux5/3 -> Bus Creator3/3  "RR CtrlOutOpt2"
  Demux4/3 -> Bus Creator2/3  "RL CtrlOutOpt2"
  Bus Creator1/1 -> Bus Creator9/2
  Demux4/2 -> Bus Creator2/2  "RL CtrlOutOpt1"
  Demux2/2 -> Bus Creator/2  "FL CtrlOutOpt1"
  Demux/2 -> Demux3/1  "FR"
  Demux3/4 -> Bus Creator1/4  "FR CtrlOutOpt3"
  Demux3/1 -> Bus Creator1/1  "FR CtrlOutOpt0"
  Demux4/4 -> Bus Creator2/4  "RL CtrlOutOpt3"
  Demux2/3 -> Bus Creator/3  "FL CtrlOutOpt2"
  Demux3/2 -> Bus Creator1/2  "FR CtrlOutOpt1"
  Demux2/1 -> Bus Creator/1  "FL CtrlOutOpt0"
  Demux3/3 -> Bus Creator1/3  "FR CtrlOutOpt2"
  In/1 -> Demux/1
  Demux5/4 -> Bus Creator3/4  "RR CtrlOutOpt3"
  Demux/3 -> Demux4/1  "RL"
  Bus Creator9/1 -> Out/1
  Demux5/2 -> Bus Creator3/2  "RR CtrlOutOpt1"
  Demux4/1 -> Bus Creator2/1  "RL CtrlOutOpt0"
  Demux/1 -> Demux2/1  "FL"

== system UserPowerTrain/CarMaker/IPG Vehicle/CarAndTrailer/Forces/Suspension Forces/CreateBus FrcSystemCtrlOutOpt ==
  note: <Your model here>
  In : Inport
  Bus Creator9 : BusCreator  Inputs=64
  Demux : Demux  Outputs=64
  Out : Outport
  wires:
  In/1 -> Demux/1
  Bus Creator9/1 -> Out/1
  Demux/64 -> Bus Creator9/64  "CtrlOutOpt63"
  Demux/1 -> Bus Creator9/1  "CtrlOutOpt0"
  Demux/2 -> Bus Creator9/2  "CtrlOutOpt1"
  Demux/3 -> Bus Creator9/3  "CtrlOutOpt2"
  Demux/4 -> Bus Creator9/4  "CtrlOutOpt3"
  Demux/5 -> Bus Creator9/5  "CtrlOutOpt4"
  Demux/6 -> Bus Creator9/6  "CtrlOutOpt5"
  Demux/7 -> Bus Creator9/7  "CtrlOutOpt6"
  Demux/8 -> Bus Creator9/8  "CtrlOutOpt7"
  Demux/9 -> Bus Creator9/9  "CtrlOutOpt8"
  Demux/10 -> Bus Creator9/10  "CtrlOutOpt9"
  Demux/11 -> Bus Creator9/11  "CtrlOutOpt10"
  Demux/12 -> Bus Creator9/12  "CtrlOutOpt11"
  Demux/13 -> Bus Creator9/13  "CtrlOutOpt12"
  Demux/14 -> Bus Creator9/14  "CtrlOutOpt13"
  Demux/15 -> Bus Creator9/15  "CtrlOutOpt14"
  Demux/16 -> Bus Creator9/16  "CtrlOutOpt15"
  Demux/17 -> Bus Creator9/17  "CtrlOutOpt16"
  Demux/18 -> Bus Creator9/18  "CtrlOutOpt17"
  Demux/19 -> Bus Creator9/19  "CtrlOutOpt18"
  Demux/20 -> Bus Creator9/20  "CtrlOutOpt19"
  Demux/21 -> Bus Creator9/21  "CtrlOutOpt20"
  Demux/22 -> Bus Creator9/22  "CtrlOutOpt21"
  Demux/23 -> Bus Creator9/23  "CtrlOutOpt22"
  Demux/24 -> Bus Creator9/24  "CtrlOutOpt23"
  Demux/25 -> Bus Creator9/25  "CtrlOutOpt24"
  Demux/26 -> Bus Creator9/26  "CtrlOutOpt25"
  Demux/27 -> Bus Creator9/27  "CtrlOutOpt26"
  Demux/28 -> Bus Creator9/28  "CtrlOutOpt27"
  Demux/29 -> Bus Creator9/29  "CtrlOutOpt28"
  Demux/30 -> Bus Creator9/30  "CtrlOutOpt29"
  Demux/31 -> Bus Creator9/31  "CtrlOutOpt30"
  Demux/32 -> Bus Creator9/32  "CtrlOutOpt31"
  Demux/33 -> Bus Creator9/33  "CtrlOutOpt32"
  Demux/34 -> Bus Creator9/34  "CtrlOutOpt33"
  Demux/35 -> Bus Creator9/35  "CtrlOutOpt34"
  Demux/36 -> Bus Creator9/36  "CtrlOutOpt35"
  Demux/37 -> Bus Creator9/37  "CtrlOutOpt36"
  Demux/38 -> Bus Creator9/38  "CtrlOutOpt37"
  Demux/39 -> Bus Creator9/39  "CtrlOutOpt38"
  Demux/40 -> Bus Creator9/40  "CtrlOutOpt39"
  Demux/41 -> Bus Creator9/41  "CtrlOutOpt40"
  Demux/42 -> Bus Creator9/42  "CtrlOutOpt41"
  Demux/43 -> Bus Creator9/43  "CtrlOutOpt42"
  Demux/44 -> Bus Creator9/44  "CtrlOutOpt43"
  Demux/45 -> Bus Creator9/45  "CtrlOutOpt44"
  Demux/46 -> Bus Creator9/46  "CtrlOutOpt45"
  Demux/47 -> Bus Creator9/47  "CtrlOutOpt46"
  Demux/48 -> Bus Creator9/48  "CtrlOutOpt47"
  Demux/49 -> Bus Creator9/49  "CtrlOutOpt48"
  Demux/50 -> Bus Creator9/50  "CtrlOutOpt49"
  Demux/51 -> Bus Creator9/51  "CtrlOutOpt50"
  Demux/52 -> Bus Creator9/52  "CtrlOutOpt51"
  Demux/53 -> Bus Creator9/53  "CtrlOutOpt52"
  Demux/54 -> Bus Creator9/54  "CtrlOutOpt53"
  Demux/55 -> Bus Creator9/55  "CtrlOutOpt54"
  Demux/56 -> Bus Creator9/56  "CtrlOutOpt55"
  Demux/57 -> Bus Creator9/57  "CtrlOutOpt56"
  Demux/58 -> Bus Creator9/58  "CtrlOutOpt57"
  Demux/59 -> Bus Creator9/59  "CtrlOutOpt58"
  Demux/60 -> Bus Creator9/60  "CtrlOutOpt59"
  Demux/61 -> Bus Creator9/61  "CtrlOutOpt60"
  Demux/62 -> Bus Creator9/62  "CtrlOutOpt61"
  Demux/63 -> Bus Creator9/63  "CtrlOutOpt62"

== system UserPowerTrain/CarMaker/IPG Vehicle/CarAndTrailer/Forces/Suspension Forces/CreateBus SpringCtrlOutOpt ==
  note: <Your model here>
  In : Inport
  Bus Creator{,1..3,9} (5 alike) : BusCreator  Inputs=4
  Demux{,2..5} (5 alike) : Demux
  Out : Outport
  wires:
  Bus Creator/1 -> Bus Creator9/1
  Demux/4 -> Demux5/1  "RR"
  Bus Creator2/1 -> Bus Creator9/3
  Demux5/1 -> Bus Creator3/1  "RR CtrlOutOpt0"
  Bus Creator3/1 -> Bus Creator9/4
  Demux2/4 -> Bus Creator/4  "FL CtrlOutOpt3"
  Demux5/3 -> Bus Creator3/3  "RR CtrlOutOpt2"
  Demux4/3 -> Bus Creator2/3  "RL CtrlOutOpt2"
  Bus Creator1/1 -> Bus Creator9/2
  Demux4/2 -> Bus Creator2/2  "RL CtrlOutOpt1"
  Demux2/2 -> Bus Creator/2  "FL CtrlOutOpt1"
  Demux/2 -> Demux3/1  "FR"
  Demux3/4 -> Bus Creator1/4  "FR CtrlOutOpt3"
  Demux3/1 -> Bus Creator1/1  "FR CtrlOutOpt0"
  Demux4/4 -> Bus Creator2/4  "RL CtrlOutOpt3"
  Demux2/3 -> Bus Creator/3  "FL CtrlOutOpt2"
  Demux3/2 -> Bus Creator1/2  "FR CtrlOutOpt1"
  Demux2/1 -> Bus Creator/1  "FL CtrlOutOpt0"
  Demux3/3 -> Bus Creator1/3  "FR CtrlOutOpt2"
  In/1 -> Demux/1
  Demux5/4 -> Bus Creator3/4  "RR CtrlOutOpt3"
  Demux/3 -> Demux4/1  "RL"
  Bus Creator9/1 -> Out/1
  Demux5/2 -> Bus Creator3/2  "RR CtrlOutOpt1"
  Demux4/1 -> Bus Creator2/1  "RL CtrlOutOpt0"
  Demux/1 -> Demux2/1  "FL"

== system UserPowerTrain/CarMaker/IPG Vehicle/CarAndTrailer/Forces/Suspension Forces/CreateBus StabiCtrlOutOpt ==
  note: <Your model here>
  In : Inport
  Bus Creator{,1..3,9} (5 alike) : BusCreator  Inputs=4
  Demux{,2..5} (5 alike) : Demux
  Out : Outport
  wires:
  Bus Creator/1 -> Bus Creator9/1
  Demux/4 -> Demux5/1  "RR"
  Bus Creator2/1 -> Bus Creator9/3
  Demux5/1 -> Bus Creator3/1  "RR CtrlOutOpt0"
  Bus Creator3/1 -> Bus Creator9/4
  Demux2/4 -> Bus Creator/4  "FL CtrlOutOpt3"
  Demux5/3 -> Bus Creator3/3  "RR CtrlOutOpt2"
  Demux4/3 -> Bus Creator2/3  "RL CtrlOutOpt2"
  Bus Creator1/1 -> Bus Creator9/2
  Demux4/2 -> Bus Creator2/2  "RL CtrlOutOpt1"
  Demux2/2 -> Bus Creator/2  "FL CtrlOutOpt1"
  Demux/2 -> Demux3/1  "FR"
  Demux3/4 -> Bus Creator1/4  "FR CtrlOutOpt3"
  Demux3/1 -> Bus Creator1/1  "FR CtrlOutOpt0"
  Demux4/4 -> Bus Creator2/4  "RL CtrlOutOpt3"
  Demux2/3 -> Bus Creator/3  "FL CtrlOutOpt2"
  Demux3/2 -> Bus Creator1/2  "FR CtrlOutOpt1"
  Demux2/1 -> Bus Creator/1  "FL CtrlOutOpt0"
  Demux3/3 -> Bus Creator1/3  "FR CtrlOutOpt2"
  In/1 -> Demux/1
  Demux5/4 -> Bus Creator3/4  "RR CtrlOutOpt3"
  Demux/3 -> Demux4/1  "RL"
  Bus Creator9/1 -> Out/1
  Demux5/2 -> Bus Creator3/2  "RR CtrlOutOpt1"
  Demux4/1 -> Bus Creator2/1  "RL CtrlOutOpt0"
  Demux/1 -> Demux2/1  "FL"

== system UserPowerTrain/CarMaker/IPG Vehicle/CarAndTrailer/Forces/Suspension Forces/CreateBus Suspension Forces ==
  note: <Your model here>
  In : Inport
  Bus Creator10 : BusCreator  Inputs=4
  Bus Creator{4..7} (4 alike) : BusCreator  Inputs=6
  Demux1 : Demux
  Demux{6..9} (4 alike) : Demux  Outputs=6
  Out : Outport
  wires:
  Demux9/5 -> Bus Creator7/5  "RR ParasiticStiffForce"
  Demux9/4 -> Bus Creator7/4  "RR BufferForce"
  Demux6/5 -> Bus Creator4/5  "FL ParasiticStiffForce"
  Demux6/6 -> Bus Creator4/6  "FL ParasiticFricForce"
  Demux1/1 -> Demux6/1  "FL"
  Demux9/1 -> Bus Creator7/1  "RR SpringForce"
  Demux9/6 -> Bus Creator7/6  "RR ParasiticFricForce"
  Demux6/4 -> Bus Creator4/4  "FL BufferForce"
  Demux8/3 -> Bus Creator6/3  "RL StabiForce"
  Demux9/2 -> Bus Creator7/2  "RR DamperForce"
  Demux8/5 -> Bus Creator6/5  "RL ParasiticStiffForce"
  Bus Creator5/1 -> Bus Creator10/2
  Bus Creator6/1 -> Bus Creator10/3
  Bus Creator4/1 -> Bus Creator10/1
  Demux8/4 -> Bus Creator6/4  "RL BufferForce"
  Demux7/1 -> Bus Creator5/1  "FR SpringForce"
  Demux8/6 -> Bus Creator6/6  "RL ParasiticFricForce"
  Demux8/2 -> Bus Creator6/2  "RL DamperForce"
  Demux1/2 -> Demux7/1  "FR"
  Demux6/2 -> Bus Creator4/2  "FL DamperForce"
  Demux1/4 -> Demux9/1  "RR"
  Demux6/1 -> Bus Creator4/1  "FL SpringForce"
  Demux8/1 -> Bus Creator6/1  "RL SpringForce"
  Demux7/3 -> Bus Creator5/3  "FR StabiForce"
  In/1 -> Demux1/1
  Demux7/6 -> Bus Creator5/6  "FR ParasiticFricForce"
  Demux6/3 -> Bus Creator4/3  "FL StabiForce"
  Demux7/2 -> Bus Creator5/2  "FR DamperForce"
  Bus Creator10/1 -> Out/1
  Demux7/5 -> Bus Creator5/5  "FR ParasiticStiffForce"
  Demux7/4 -> Bus Creator5/4  "FR BufferForce"
  Demux9/3 -> Bus Creator7/3  "RR StabiForce"
  Demux1/3 -> Demux8/1  "RL"
  Bus Creator7/1 -> Bus Creator10/4

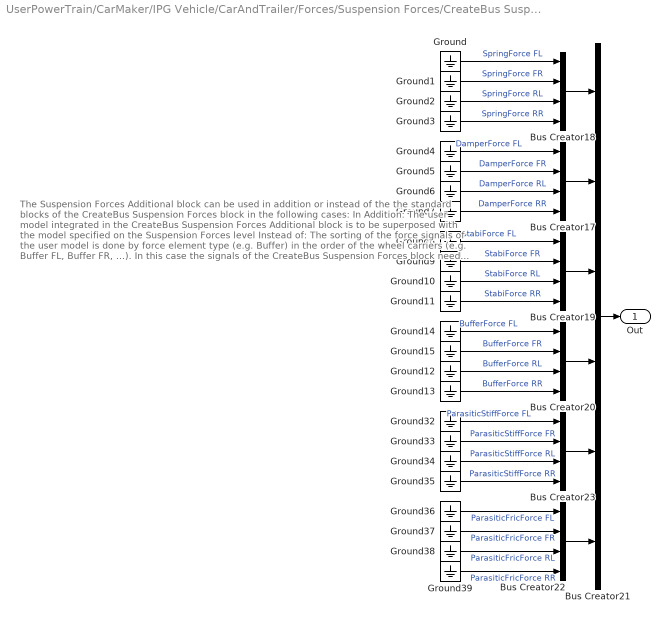
== system UserPowerTrain/CarMaker/IPG Vehicle/CarAndTrailer/Forces/Suspension Forces/CreateBus Suspension Forces Additional ==
  note: The Suspension Forces Additional block can be used in addition or instead of the
      | the standard blocks of the CreateBus Suspension Forces block in the following cases:
      |
      | In Addition: The user model integrated in the CreateBus Suspension Forces Additional block is to be superposed with the model specified on the Suspension Forces level
      | Instead of: The sorting of the force signals of the user model is done by force element type (e.g. Buffer) in the order of the wheel carriers (e.g. Buffer FL, Buffer FR, ...). In this case the signals of the CreateBus Suspension Forces block need to be disabled e.g. by manually connecting them to ground signals.
      |
      | ATTENTION : The forces given in the CreateBus Suspension Forces Additional block are internally added to the forces of the Suspension Forces block. If this is not desired, make sure to include a force model only in one of the two levels.
  Bus Creator{17..20,22..23} (6 alike) : BusCreator  Inputs=4
  Bus Creator21 : BusCreator  Inputs=6
  Ground{,1..15,32..39} (24 alike) : Ground
  Out : Outport
  wires:
  Ground1/1 -> Bus Creator18/2  "SpringForce FR"
  Ground9/1 -> Bus Creator19/2  "StabiForce FR"
  Ground8/1 -> Bus Creator19/1  "StabiForce FL"
  Bus Creator22/1 -> Bus Creator21/6
  Bus Creator21/1 -> Out/1
  Ground/1 -> Bus Creator18/1  "SpringForce FL"
  Ground36/1 -> Bus Creator22/1  "ParasiticFricForce FL"
  Ground2/1 -> Bus Creator18/3  "SpringForce RL"
  Ground5/1 -> Bus Creator17/2  "DamperForce FR"
  Ground15/1 -> Bus Creator20/2  "BufferForce FR"
  Ground35/1 -> Bus Creator23/4  "ParasiticStiffForce RR"
  Bus Creator20/1 -> Bus Creator21/4
  Bus Creator17/1 -> Bus Creator21/2
  Ground37/1 -> Bus Creator22/2  "ParasiticFricForce FR"
  Ground4/1 -> Bus Creator17/1  "DamperForce FL"
  Ground33/1 -> Bus Creator23/2  "ParasiticStiffForce FR"
  Bus Creator23/1 -> Bus Creator21/5
  Ground11/1 -> Bus Creator19/4  "StabiForce RR"
  Ground10/1 -> Bus Creator19/3  "StabiForce RL"
  Ground6/1 -> Bus Creator17/3  "DamperForce RL"
  Bus Creator19/1 -> Bus Creator21/3
  Ground7/1 -> Bus Creator17/4  "DamperForce RR"
  Bus Creator18/1 -> Bus Creator21/1
  Ground34/1 -> Bus Creator23/3  "ParasiticStiffForce RL"
  Ground3/1 -> Bus Creator18/4  "SpringForce RR"
  Ground12/1 -> Bus Creator20/3  "BufferForce RL"
  Ground38/1 -> Bus Creator22/3  "ParasiticFricForce RL"
  Ground14/1 -> Bus Creator20/1  "BufferForce FL"
  Ground39/1 -> Bus Creator22/4  "ParasiticFricForce RR"
  Ground32/1 -> Bus Creator23/1  "ParasiticStiffForce FL"
  Ground13/1 -> Bus Creator20/4  "BufferForce RR"

== system UserPowerTrain/CarMaker/IPG Vehicle/CarAndTrailer/Forces/Suspension Forces/CreateBus Suspension Forces CtrlOut ==
  note: <Your model here>
  In : Inport
  Bus Creator{,1..3,9} (5 alike) : BusCreator  Inputs=4
  Demux{,2..5} (5 alike) : Demux
  Out : Outport
  wires:
  Bus Creator3/1 -> Bus Creator9/4
  Demux2/4 -> Bus Creator/4  "FL BufferCtrlOut"
  Demux/4 -> Demux5/1  "RR"
  Bus Creator2/1 -> Bus Creator9/3
  Demux3/1 -> Bus Creator1/1  "FR SpringCtrlOut"
  Bus Creator/1 -> Bus Creator9/1
  Demux5/1 -> Bus Creator3/1  "RR SpringCtrlOut"
  Demux5/2 -> Bus Creator3/2  "RR DamperCtrlOut"
  Demux4/2 -> Bus Creator2/2  "RL DamperCtrlOut"
  Demux4/3 -> Bus Creator2/3  "RL StabiCtrlOut"
  Demux2/2 -> Bus Creator/2  "FL DamperCtrlOut"
  Demux/3 -> Demux4/1  "RL"
  Demux5/4 -> Bus Creator3/4  "RR BufferCtrlOut"
  In/1 -> Demux/1
  Demux2/1 -> Bus Creator/1  "FL SpringCtrlOut"
  Demux3/3 -> Bus Creator1/3  "FR StabiCtrlOut"
  Demux3/2 -> Bus Creator1/2  "FR DamperCtrlOut"
  Demux4/1 -> Bus Creator2/1  "RL SpringCtrlOut"
  Demux4/4 -> Bus Creator2/4  "RL BufferCtrlOut"
  Demux2/3 -> Bus Creator/3  "FL StabiCtrlOut"
  Bus Creator1/1 -> Bus Creator9/2
  Bus Creator9/1 -> Out/1
  Demux/1 -> Demux2/1  "FL"
  Demux/2 -> Demux3/1  "FR"
  Demux5/3 -> Bus Creator3/3  "RR StabiCtrlOut"
  Demux3/4 -> Bus Creator1/4  "FR BufferCtrlOut"

== system UserPowerTrain/CarMaker/IPG Vehicle/CarAndTrailer/Forces/Suspension Forces/Damper CreateBus CtrlOutOpt ==
  note: <Your model here>
  In : Inport
  Bus Creator{,1..3,9} (5 alike) : BusCreator  Inputs=4
  Demux{,2..5} (5 alike) : Demux
  Out : Outport
  wires:
  Bus Creator/1 -> Bus Creator9/1
  Demux/4 -> Demux5/1  "RR"
  Bus Creator2/1 -> Bus Creator9/3
  Demux5/1 -> Bus Creator3/1  "RR CtrlOutOpt0"
  Bus Creator3/1 -> Bus Creator9/4
  Demux2/4 -> Bus Creator/4  "FL CtrlOutOpt3"
  Demux5/3 -> Bus Creator3/3  "RR CtrlOutOpt2"
  Demux4/3 -> Bus Creator2/3  "RL CtrlOutOpt2"
  Bus Creator1/1 -> Bus Creator9/2
  Demux4/2 -> Bus Creator2/2  "RL CtrlOutOpt1"
  Demux2/2 -> Bus Creator/2  "FL CtrlOutOpt1"
  Demux/2 -> Demux3/1  "FR"
  Demux3/4 -> Bus Creator1/4  "FR CtrlOutOpt3"
  Demux3/1 -> Bus Creator1/1  "FR CtrlOutOpt0"
  Demux4/4 -> Bus Creator2/4  "RL CtrlOutOpt3"
  Demux2/3 -> Bus Creator/3  "FL CtrlOutOpt2"
  Demux3/2 -> Bus Creator1/2  "FR CtrlOutOpt1"
  Demux2/1 -> Bus Creator/1  "FL CtrlOutOpt0"
  Demux3/3 -> Bus Creator1/3  "FR CtrlOutOpt2"
  In/1 -> Demux/1
  Demux5/4 -> Bus Creator3/4  "RR CtrlOutOpt3"
  Demux/3 -> Demux4/1  "RL"
  Bus Creator9/1 -> Out/1
  Demux5/2 -> Bus Creator3/2  "RR CtrlOutOpt1"
  Demux4/1 -> Bus Creator2/1  "RL CtrlOutOpt0"
  Demux/1 -> Demux2/1  "FL"

== system UserPowerTrain/CarMaker/IPG Vehicle/CarAndTrailer/Forces/Suspension Forces/FrcSystem CreateBus CtrlOutOpt ==
  note: <Your model here>
  In : Inport
  Bus Creator9 : BusCreator  Inputs=64
  Demux : Demux  Outputs=64
  Out : Outport
  wires:
  In/1 -> Demux/1
  Bus Creator9/1 -> Out/1
  Demux/64 -> Bus Creator9/64  "CtrlOutOpt63"
  Demux/1 -> Bus Creator9/1  "CtrlOutOpt0"
  Demux/2 -> Bus Creator9/2  "CtrlOutOpt1"
  Demux/3 -> Bus Creator9/3  "CtrlOutOpt2"
  Demux/4 -> Bus Creator9/4  "CtrlOutOpt3"
  Demux/5 -> Bus Creator9/5  "CtrlOutOpt4"
  Demux/6 -> Bus Creator9/6  "CtrlOutOpt5"
  Demux/7 -> Bus Creator9/7  "CtrlOutOpt6"
  Demux/8 -> Bus Creator9/8  "CtrlOutOpt7"
  Demux/9 -> Bus Creator9/9  "CtrlOutOpt8"
  Demux/10 -> Bus Creator9/10  "CtrlOutOpt9"
  Demux/11 -> Bus Creator9/11  "CtrlOutOpt10"
  Demux/12 -> Bus Creator9/12  "CtrlOutOpt11"
  Demux/13 -> Bus Creator9/13  "CtrlOutOpt12"
  Demux/14 -> Bus Creator9/14  "CtrlOutOpt13"
  Demux/15 -> Bus Creator9/15  "CtrlOutOpt14"
  Demux/16 -> Bus Creator9/16  "CtrlOutOpt15"
  Demux/17 -> Bus Creator9/17  "CtrlOutOpt16"
  Demux/18 -> Bus Creator9/18  "CtrlOutOpt17"
  Demux/19 -> Bus Creator9/19  "CtrlOutOpt18"
  Demux/20 -> Bus Creator9/20  "CtrlOutOpt19"
  Demux/21 -> Bus Creator9/21  "CtrlOutOpt20"
  Demux/22 -> Bus Creator9/22  "CtrlOutOpt21"
  Demux/23 -> Bus Creator9/23  "CtrlOutOpt22"
  Demux/24 -> Bus Creator9/24  "CtrlOutOpt23"
  Demux/25 -> Bus Creator9/25  "CtrlOutOpt24"
  Demux/26 -> Bus Creator9/26  "CtrlOutOpt25"
  Demux/27 -> Bus Creator9/27  "CtrlOutOpt26"
  Demux/28 -> Bus Creator9/28  "CtrlOutOpt27"
  Demux/29 -> Bus Creator9/29  "CtrlOutOpt28"
  Demux/30 -> Bus Creator9/30  "CtrlOutOpt29"
  Demux/31 -> Bus Creator9/31  "CtrlOutOpt30"
  Demux/32 -> Bus Creator9/32  "CtrlOutOpt31"
  Demux/33 -> Bus Creator9/33  "CtrlOutOpt32"
  Demux/34 -> Bus Creator9/34  "CtrlOutOpt33"
  Demux/35 -> Bus Creator9/35  "CtrlOutOpt34"
  Demux/36 -> Bus Creator9/36  "CtrlOutOpt35"
  Demux/37 -> Bus Creator9/37  "CtrlOutOpt36"
  Demux/38 -> Bus Creator9/38  "CtrlOutOpt37"
  Demux/39 -> Bus Creator9/39  "CtrlOutOpt38"
  Demux/40 -> Bus Creator9/40  "CtrlOutOpt39"
  Demux/41 -> Bus Creator9/41  "CtrlOutOpt40"
  Demux/42 -> Bus Creator9/42  "CtrlOutOpt41"
  Demux/43 -> Bus Creator9/43  "CtrlOutOpt42"
  Demux/44 -> Bus Creator9/44  "CtrlOutOpt43"
  Demux/45 -> Bus Creator9/45  "CtrlOutOpt44"
  Demux/46 -> Bus Creator9/46  "CtrlOutOpt45"
  Demux/47 -> Bus Creator9/47  "CtrlOutOpt46"
  Demux/48 -> Bus Creator9/48  "CtrlOutOpt47"
  Demux/49 -> Bus Creator9/49  "CtrlOutOpt48"
  Demux/50 -> Bus Creator9/50  "CtrlOutOpt49"
  Demux/51 -> Bus Creator9/51  "CtrlOutOpt50"
  Demux/52 -> Bus Creator9/52  "CtrlOutOpt51"
  Demux/53 -> Bus Creator9/53  "CtrlOutOpt52"
  Demux/54 -> Bus Creator9/54  "CtrlOutOpt53"
  Demux/55 -> Bus Creator9/55  "CtrlOutOpt54"
  Demux/56 -> Bus Creator9/56  "CtrlOutOpt55"
  Demux/57 -> Bus Creator9/57  "CtrlOutOpt56"
  Demux/58 -> Bus Creator9/58  "CtrlOutOpt57"
  Demux/59 -> Bus Creator9/59  "CtrlOutOpt58"
  Demux/60 -> Bus Creator9/60  "CtrlOutOpt59"
  Demux/61 -> Bus Creator9/61  "CtrlOutOpt60"
  Demux/62 -> Bus Creator9/62  "CtrlOutOpt61"
  Demux/63 -> Bus Creator9/63  "CtrlOutOpt62"
